simulink model "simu"  (R2025b)
settings: Solver=FixedStepAuto  StartTime=0.0  StopTime=25  FixedStep=0.01  RelTol=1e-3
InitFcn:
  | load("Scheduledata.mat")
model workspace (MAT data in the model file):
  T_data = [16.81; 22.34; 22.23; 21.49; 20; 20.21; 18.09; 15.74; 13.4; 10.85; 10.21; 8.94; 8.83; 8.62; 8.62; 8.62; 8.51; 8.72; 8.51; 8.51; 7.77; 7.02; 5.64; 3.83; 2.23; 0.96; 0]
  aero_data.Alpha = [0; 2; 4]
  aero_data.CD = [0.20580088598; 0.20580088598; 0.20580088598]
  aero_data.CL = [0; 0.0625795358549; 0.124860076206]
  aero_data.CP = [0.999; 0.999; 0.999]
  t_data = [0.01; 0.03; 0.11; 0.26; 0.37; 0.47; 0.67; 0.99; 1.31; 1.81; 2.49; 3.13; 3.6; 4.11; 4.95; 5.45; 5.58; 5.88; 6.22; 6.46; 6.6; 6.71; 6.79; 6.91; 6.95; 7; 7.05]
values from neighbouring files (symbols this model uses):
  q = logsout.get('q').Values    [run_nominal.m]
undefined symbols (not defined in the file or in its folder): F, Light, MIL
libraries: simulink_extras x3, aerolibwind2 x1, aerolibatmos2 x1
settings Model: Creator=arjun  LastModifiedBy=zachm
settings DataIOCC: DatasetSignalFormat=timetable

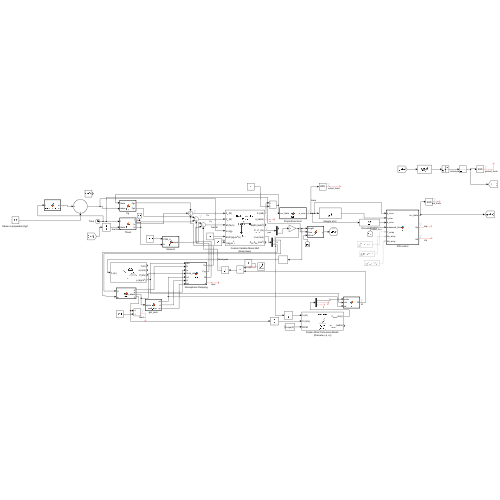
[thumbnail: Simulink's stored preview of the top-level diagram]
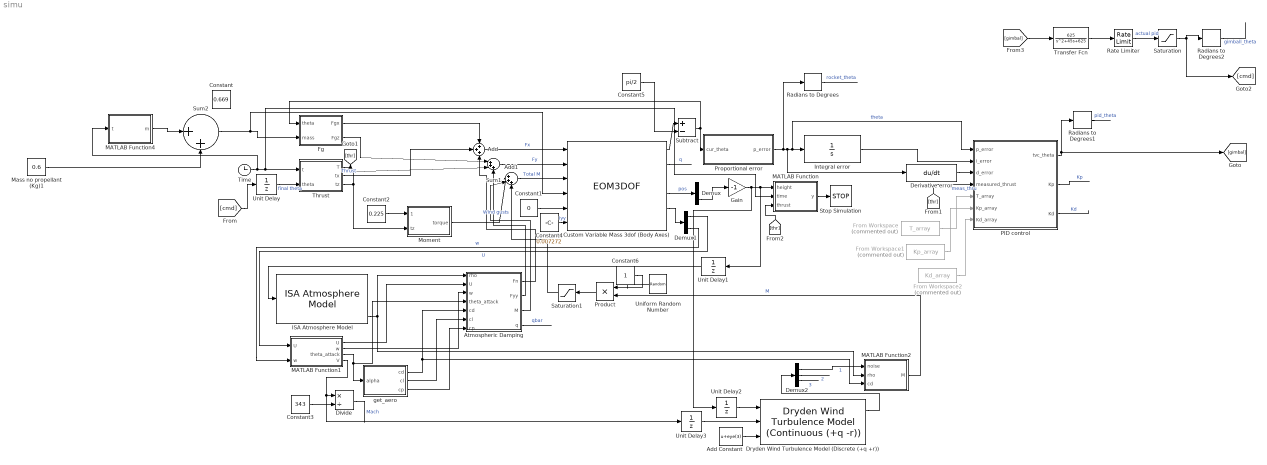
== system simu ==
  Add : Sum  Inputs=+++
  Add Constant : Bias  Bias=eye(3)  SaturateOnIntegerOverflow=off
  Add1 : Sum  Inputs=|+++
  Atmospheric Damping : MATLAB Function  TreatAsAtomicUnit=on
  Constant : Constant  Value=0.669
  Constant1 : Constant  Value=0
  Constant2 : Constant  Value=0.225
  Constant3 : Constant  Value=343
  Constant4 : Constant  Value=0.007272  VectorParams1D=off
  Constant5 : Constant  Value=pi/2
  Constant6 : Constant
  Custom Variable Mass 3dof (Body Axes) : EOM3DOF  mtype=Custom Variable  v_ini=.01  theta_ini=deg2rad(93)  g=0
  Demux : Demux  Outputs=2
  Demux1 : Demux  Outputs=2
  Demux2 : Demux  Outputs=3
  Derivative error : Derivative
  Divide : Product  Inputs=*/
  Dryden Wind Turbulence Model (Discrete (+q +r)) : aerolibwind2/Dryden Wind Turbulence Model  (Continuous (+q -r))  units=Metric (MKS)  spec=MIL-F-8785C  model=Discrete Dryden (+q +r)  W20=15  Wdeg=0  TurbProb=10^-2 - Light  L_high=533.4  Wingspan=10  ts=0.1  Seed=randi(10000, 1, 4)  T_on=on
      settings: LibrarySourceBlock=|
      | aerolibwind2/Dryden Wind Turbulence Model
      | (Discrete (+q +r))
  Fg : MATLAB Function  TreatAsAtomicUnit=on
  From Workspace : FromWorkspace  Commented=on  VariableName=T_array  SampleTime=-1  Interpolate=off  OutputAfterFinalValue=Holding final value
  From Workspace1 : FromWorkspace  Commented=on  VariableName=Kp_array  SampleTime=-1
  From Workspace2 : FromWorkspace  Commented=on  VariableName=Kd_array  SampleTime=-1
  Gain : Gain  Gain=-1
  ISA Atmosphere Model : aerolibatmos2/ISA Atmosphere Model  useExtended=off  action=Warning  custom=off  viscosityOut=off  g=9.80665  gamma=1.4  R=287.0531  L=0.0065  h_trop=11000  h_strat=20000  rho0=1.225  P0=101325  T0=288.15  h0=0  S=110.4  Tref=273.15  muref=1.716e-5
  Integral error : Integrator  LimitOutput=on  UpperSaturationLimit=0.5  LowerSaturationLimit=-0.5  ContinuousStateAttributes='error'
  MATLAB Function : MATLAB Function  TreatAsAtomicUnit=on
  MATLAB Function1 : MATLAB Function  TreatAsAtomicUnit=on
  MATLAB Function2 : MATLAB Function  TreatAsAtomicUnit=on
  MATLAB Function4 : MATLAB Function  TreatAsAtomicUnit=on
  Mass no propellant (Kg)1 : Constant  Value=0.6
  Moment : MATLAB Function  TreatAsAtomicUnit=on
  PID control : MATLAB Function  TreatAsAtomicUnit=on
  Product : Product
  Proportional error : MATLAB Function  TreatAsAtomicUnit=on
  Radians to Degrees : simulink_extras/Transformations/Radians to Degrees
  Radians to Degrees1 : simulink_extras/Transformations/Radians to Degrees
  Radians to Degrees2 : simulink_extras/Transformations/Radians to Degrees
  Rate Limiter : RateLimiter  RisingSlewLimit=5  FallingSlewLimit=-5  SampleTimeMode=inherited
  Saturation : Saturate  UpperLimit=0.1  LowerLimit=-0.1
  Saturation1 : Saturate  UpperLimit=.01  LowerLimit=-0.01
  Stop Simulation : Stop
  Subtract : Sum  Inputs=+-
  Sum1 : Sum  Inputs=|+++
  Sum2 : Sum  Inputs=|++
  Thrust : MATLAB Function  TreatAsAtomicUnit=on
  Time : Clock
  Transfer Fcn : TransferFcn  Numerator=625  Denominator=[1 45 625]
  Uniform Random Number : UniformRandomNumber  Seed=randi(1000)  SampleTime=1
  Unit Delay{,1..3} (4 alike) : UnitDelay  SampleTime=-1  HasFrameUpgradeWarning=on
  get_aero : MATLAB Function  TreatAsAtomicUnit=on
  wires:
  Fg/2(Fgz) -> Sum1/1
  Thrust/3(tz) -> Moment/2(tz), Sum1/2
  Sum1/1 -> Custom Variable Mass 3dof (Body Axes)/2  "Fy"
  Add/1 -> Custom Variable Mass 3dof (Body Axes)/1  "Fx"
  Custom Variable Mass 3dof (Body Axes)/4 -> Demux/1  "pos"
  Constant4/1 -> Custom Variable Mass 3dof (Body Axes)/6  "Iyy"
  Derivative error/1 -> PID control/3(d_error)
  Integral error/1 -> PID control/2(i_error)
  Proportional error/1(p_error) -> Integral error/1, PID control/1(p_error), Derivative error/1, Radians to Degrees/1  "theta"
  Constant1/1 -> Custom Variable Mass 3dof (Body Axes)/5
  Radians to Degrees/1 -> ?  "rocket_theta"
  Radians to Degrees1/1 -> ?  "pid_theta"
  Fg/1(Fgx) -> Add/1
  Thrust/2(tx) -> Add/2
  Constant2/1 -> Moment/1(COM_d)
  Demux/2 -> Gain/1
  MATLAB Function/1(y) -> Stop Simulation/1
  Custom Variable Mass 3dof (Body Axes)/5 -> Demux1/1
  Demux1/1 -> MATLAB Function1/1("U ")  "U"
  Demux1/2 -> MATLAB Function1/2("w ")  "w"
  MATLAB Function1/1(U) -> Atmospheric Damping/2(U)
  MATLAB Function1/2(w) -> Atmospheric Damping/3(w)
  ISA Atmosphere Model/4 -> Atmospheric Damping/1(rho), MATLAB Function2/2(rho)
  Moment/1(torque) -> Add1/1
  Add1/1 -> Custom Variable Mass 3dof (Body Axes)/3  "Total M"
  MATLAB Function1/3(theta_attack) -> get_aero/1(alpha), Atmospheric Damping/4(theta_attack)
  get_aero/1(cd) -> Atmospheric Damping/5(cd), MATLAB Function2/3(cd)
  get_aero/2(cl) -> Atmospheric Damping/6(cl)
  get_aero/3(cp) -> Atmospheric Damping/7(cp)
  PID control/1(tvc_theta) -> Radians to Degrees1/1, [gimbal]
  Gain/1 -> Unit Delay2/1, MATLAB Function/1(height), Unit Delay1/1
  [cmd] -> Unit Delay/1
  Custom Variable Mass 3dof (Body Axes)/1 -> Subtract/1
  Constant5/1 -> Subtract/2
  Subtract/1 -> Fg/1(theta), Proportional error/1(cur_theta)
  Atmospheric Damping/1(Fn) -> Add/3
  Atmospheric Damping/2(Fyy) -> Sum1/3
  Atmospheric Damping/3(M) -> Add1/2
  Unit Delay1/1 -> ISA Atmosphere Model/1
  Thrust/1(T) -> [thr]  "Thrust"
  Custom Variable Mass 3dof (Body Axes)/2 -> ?  "q"
  Atmospheric Damping/4(q) -> ?  "qbar"
  MATLAB Function1/4(V) -> Unit Delay3/1, Divide/1
  Constant3/1 -> Divide/2
  Divide/1 -> ?  "Mach"
  [thr] -> PID control/4(measured_thrust)  "meas_thru"
  From Workspace/1 -> PID control/5(T_array)
  From Workspace1/1 -> PID control/6(Kp_array)
  From Workspace2/1 -> PID control/7(Kd_array)
  Add Constant/1 -> Dryden Wind Turbulence Model (Discrete (+q +r))/3
  Dryden Wind Turbulence Model (Discrete (+q +r))/1 -> Demux2/1
  Demux2/1 -> MATLAB Function2/1(noise)  "1"
  Demux2/3 -> ?  "3"
  Demux2/2 -> ?  "2"
  Unit Delay2/1 -> Dryden Wind Turbulence Model (Discrete (+q +r))/1
  Unit Delay3/1 -> Dryden Wind Turbulence Model (Discrete (+q +r))/2
  MATLAB Function2/1(M) -> Product/2  "M"
  [thr] -> MATLAB Function/3(thrust)
  PID control/2(Kp) -> ?  "Kp"
  PID control/3(Kd) -> ?  "Kd"
  Radians to Degrees2/1 -> ?  "gimball_theta"
  Uniform Random Number/1 -> ?
  Product/1 -> Saturation1/1
  Transfer Fcn/1 -> Rate Limiter/1
  Rate Limiter/1 -> Saturation/1  "actual pid"
  Saturation/1 -> [cmd], Radians to Degrees2/1
  [gimbal] -> Transfer Fcn/1
  Unit Delay/1 -> Thrust/2(theta)  "final theta"
  Constant6/1 -> Product/1
  Saturation1/1 -> Add1/3  "Wind gusts"
  MATLAB Function4/1(m) -> Sum2/1
  Mass no propellant (Kg)1/1 -> Sum2/2
  Time/1 -> MATLAB Function4/1(t), MATLAB Function/2(time), Thrust/1(t)
  Sum2/1 -> Custom Variable Mass 3dof (Body Axes)/4, Fg/2(mass)

== matlab function simu/get_aero ==
  data: alpha input; cd output; cl output; cp output
function [cd, cl, cp] = get_aero(alpha)

    S = load("alpha_interp.mat");  
    Alpha = S.aero_data.Alpha;
    CD_full = S.aero_data.CD;
    CL_full = S.aero_data.CL;
    CP_full = S.aero_data.CP;

    cd = interp1(Alpha, CD_full, alpha, 'linear', 'extrap');
    cl = interp1(Alpha, CL_full, alpha, 'linear', 'extrap');
    cp = interp1(Alpha, CP_full, alpha, 'linear', 'extrap');
    cp = cp * 0.3048;
end

== matlab function simu/MATLAB Function2 ==
  data: noise input; M output; rho input; cd input
function M = fcn(noise, rho, cd)
A = 0.079 * 0.762;
F = 1/2 * noise^2 * rho * cd * A;
M = 0.225 * F;

== matlab function simu/MATLAB Function4 ==
  data: t input; m output
function m = propellantmass(t)
    %#codegen
    m = ((0.3567 * t^2) - (8.072 *t) + 39.18)/1000;
    end

== matlab function simu/Moment ==
  data: COM_d input; torque output; tz input
function torque = fcn(COM_d, tz)

torque = COM_d * tz;

== matlab function simu/Thrust ==
  data: T output; t input; tx output; tz output; theta input
function [T, tx, tz] = fcn(t, theta)
    persistent thrust_interp;
    
    if isempty(thrust_interp)
        loadedData = load('interp_thrust_data.mat'); 
        disp(loadedData)
        t_data = loadedData.t_data;
        T_data = loadedData.T_data; 

        thrust_interp = @(t) interp1(t_data, T_data, t, 'pchip', 'extrap');
    end

    burnout_time = 7.05;
    if t < burnout_time
        T = thrust_interp(t);
    else
        T = 0;
    end
    
    tx = T * cos(theta);
    tz = -T * sin(theta);
end

== matlab function simu/MATLAB Function ==
  data: height input; time input; y output; thrust input
function y = fcn(height, time, thrust)

if (time > 1 && height < 0) || (time > 1 && thrust <= 0)
    y = 1;
else
    y = 0;
end

== matlab function simu/Fg ==
  data: theta input; mass input; Fgx output; Fgz output
function [Fgx, Fgz]= fcn(theta, mass)

Fgx = mass * -cos(theta) * 9.8;
Fgz = mass * sin(theta) * -9.8;

== matlab function simu/Proportional error ==
  data: cur_theta input; p_error output
function p_error = fcn(cur_theta)
    p_error = cur_theta;
end

== matlab function simu/PID control ==
  data: p_error input; tvc_theta output; i_error input; d_error input; measured_thrust input; T_array input; Kp_array input; Kd_array input; Kp output; Kd output
function [tvc_theta, Kp, Kd] = fcn(p_error, i_error, d_error, measured_thrust, T_array, Kp_array, Kd_array)
    
    %     loadedSchedule = load('interp_thrust_data.mat'); 
    
    T_array = [0, 9, 11, 24];
    Kp_array = [0.19, 0.15, 0.13, 0.1];
    Kd_array = [0.05, 0.04, 0.03, 0.02];
    T_current = measured_thrust;
    
    Kp = interp1(T_array, Kp_array, T_current, 'linear', 'extrap');
    Kd = interp1(T_array, Kd_array, T_current, 'linear', 'extrap');
    Kd = 0.3* Kp;
    Ki = 0;

    tvc_theta = Kp * p_error + Ki * i_error + Kd * d_error;
    tvc_theta = max(min(tvc_theta, deg2rad(7)), -deg2rad(7));
end

== matlab function simu/MATLAB Function1 ==
  data: U output; w output; U input; w input; theta_attack output; V output
function [U, w, theta_attack, V] = fcn(U, w)

theta_attack = atan(w/U);
V = sqrt(U^2 + w^2);

== matlab function simu/Atmospheric Damping ==
  data: rho input; Fn output; U input; w input; theta_attack input; cd input; cl input; cp input; Fyy output; M output; q output
function [Fn, Fyy, M, q] = fcn(rho, U, w, theta_attack, cd, cl, cp)
    V = sqrt(U^2 + w^2);

    Sref = pi * (0.0762/2)^2;

    q = 1/2 * rho * V^2;

    L = q * cl * Sref;
    D = q * cd * Sref;

    Xw = -D;
    Zw = -L;
    
    cg = 0.3302; % from nosecone

    Fn =  cos(theta_attack)*Xw - sin(theta_attack)*Zw
    Fyy =  sin(theta_attack)*Xw + cos(theta_attack)*Zw
    M = Fyy * (cp - cg);
end
